simulink model "TEST2_Thermostat_Logic"  (R2025b)
settings: Solver=FixedStepAuto  StartTime=0.0  StopTime=60  FixedStep=0.1  RelTol=1e-3
settings Model: Creator=daniel.camacho  LastModifiedBy=daniel.camacho

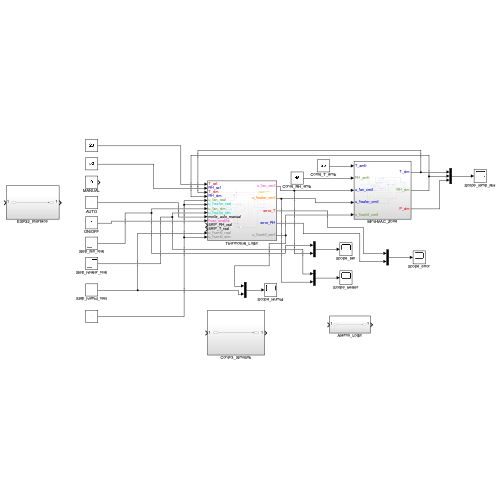
[thumbnail: Simulink's stored preview of the top-level diagram]
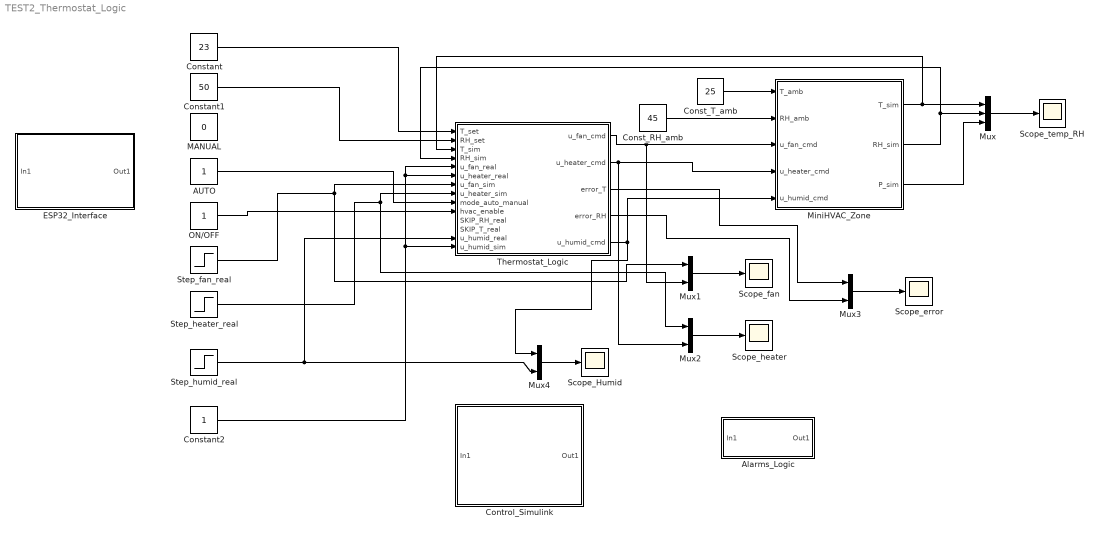
== system TEST2_Thermostat_Logic ==
  AUTO : Constant
  Alarms_Logic : Subsystem
  Const_RH_amb : Constant  Value=45
  Const_T_amb : Constant  Value=25
  Constant : Constant  Value=23
  Constant1 : Constant  Value=50
  Constant2 : Constant
  Control_Simulink : Subsystem
  ESP32_Interface : Subsystem
  MANUAL : Constant  Value=0
  MiniHVAC_Zone : Subsystem
  Mux : Mux  Inputs=3
  Mux{1..4} (4 alike) : Mux  Inputs=2
  ON/OFF : Constant
  Scope_Humid : Scope
      settings: ActiveDisplayYMinimum=-0.12499999999999997  ActiveDisplayYMaximum=1.125  DataLoggingVariableName=ScopeData3
  Scope_error : Scope
      settings: ActiveDisplayYMinimum=-2.875  ActiveDisplayYMaximum=5.875  DataLoggingVariableName=ScopeData4
  Scope_fan : Scope
      settings: ActiveDisplayYMinimum=-0.19683069160090955  ActiveDisplayYMaximum=1.476509953511558
  Scope_heater : Scope
      settings: ActiveDisplayYMinimum=-0.12499999999999997  ActiveDisplayYMaximum=1.125  DataLoggingVariableName=ScopeData2
  Scope_temp_RH : Scope
      settings: ActiveDisplayYMinimum=-1  ActiveDisplayYMaximum=1
  Step_fan_real : Step  Time=10  SampleTime=0
  Step_heater_real : Step  Time=20  SampleTime=0
  Step_humid_real : Step  Time=10  SampleTime=0
  Thermostat_Logic : Subsystem
  wires:
  Constant/1 -> Thermostat_Logic/1(T_set)
  Constant1/1 -> Thermostat_Logic/2(RH_set)
  ON/OFF/1 -> Thermostat_Logic/10(hvac_enable)
  Step_fan_real/1 -> Thermostat_Logic/7(u_fan_sim), Mux1/1
  Step_heater_real/1 -> Thermostat_Logic/8(u_heater_sim), Mux2/1
  Constant2/1 -> Thermostat_Logic/14(u_humid_sim), Thermostat_Logic/6(u_heater_real), Thermostat_Logic/5(u_fan_real)
  MiniHVAC_Zone/1(T_sim) -> Mux/1, Thermostat_Logic/3(T_sim)
  MiniHVAC_Zone/2(RH_sim) -> Mux/2, Thermostat_Logic/4(RH_sim)
  Thermostat_Logic/1(u_fan_cmd) -> MiniHVAC_Zone/3(u_fan_cmd), Mux1/2
  Thermostat_Logic/2(u_heater_cmd) -> MiniHVAC_Zone/4(u_heater_cmd), Mux2/2
  Const_T_amb/1 -> MiniHVAC_Zone/1(T_amb)
  Const_RH_amb/1 -> MiniHVAC_Zone/2(RH_amb)
  Mux/1 -> Scope_temp_RH/1
  MiniHVAC_Zone/3(P_sim) -> Mux/3
  Mux1/1 -> Scope_fan/1
  Mux2/1 -> Scope_heater/1
  Mux3/1 -> Scope_error/1
  Thermostat_Logic/3(error_T) -> Mux3/1
  Thermostat_Logic/4(error_RH) -> Mux3/2
  AUTO/1 -> Thermostat_Logic/9(mode_auto_manual)
  Mux4/1 -> Scope_Humid/1
  Step_humid_real/1 -> Thermostat_Logic/13(u_humid_real), Mux4/2
  Thermostat_Logic/5(u_humid_cmd) -> Mux4/1, MiniHVAC_Zone/5(u_humid_cmd)

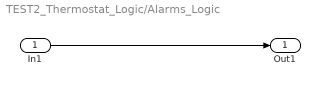
== system TEST2_Thermostat_Logic/Alarms_Logic ==
  In1 : Inport
  Out1 : Outport
  wires:
  In1/1 -> Out1/1

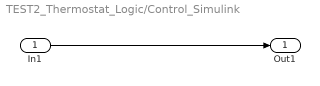
== system TEST2_Thermostat_Logic/Control_Simulink ==
  In1 : Inport
  Out1 : Outport
  wires:
  In1/1 -> Out1/1

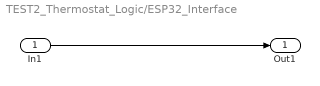
== system TEST2_Thermostat_Logic/ESP32_Interface ==
  In1 : Inport
  Out1 : Outport
  wires:
  In1/1 -> Out1/1

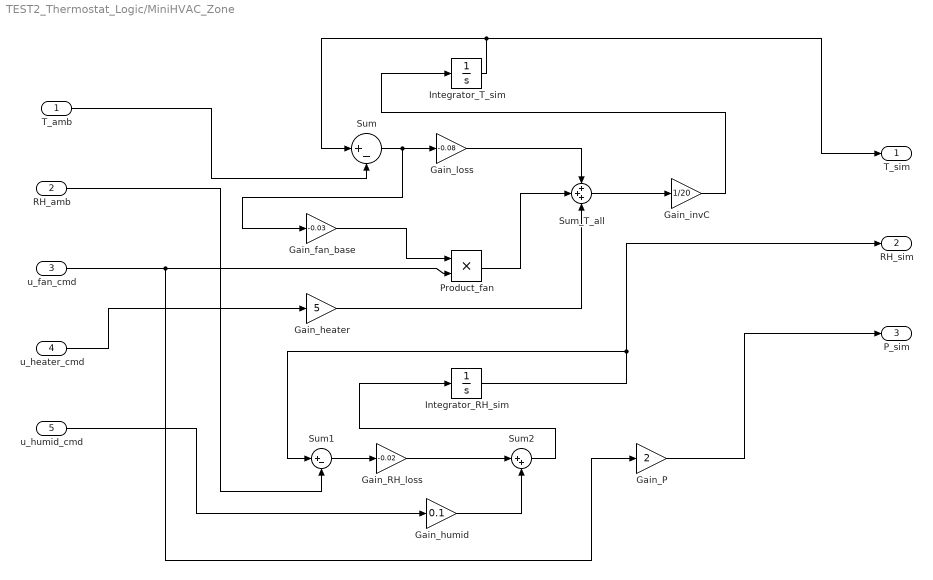
== system TEST2_Thermostat_Logic/MiniHVAC_Zone ==
  T_amb : Inport
  RH_amb : Inport  Port=2
  u_fan_cmd : Inport  Port=3
  u_heater_cmd : Inport  Port=4
  u_humid_cmd : Inport  Port=5
  Gain_P : Gain  Gain=2
  Gain_RH_loss : Gain  Gain=-0.02
  Gain_fan_base : Gain  Gain=-0.03
  Gain_heater : Gain  Gain=5
  Gain_humid : Gain  Gain=0.1
  Gain_invC : Gain  Gain=1/20
  Gain_loss : Gain  Gain=-0.08
  Integrator_RH_sim : Integrator  InitialCondition=45
  Integrator_T_sim : Integrator  InitialCondition=25
  Product_fan : Product
  Sum : Sum  Inputs=|+-
  Sum1 : Sum  Inputs=|+-
  Sum2 : Sum  Inputs=|++
  Sum_T_all : Sum  Inputs=+++
  T_sim : Outport
  RH_sim : Outport  Port=2
  P_sim : Outport  Port=3
  wires:
  Integrator_T_sim/1 -> T_sim/1, Sum/1
  T_amb/1 -> Sum/2
  Gain_fan_base/1 -> Product_fan/1
  u_fan_cmd/1 -> Gain_P/1, Product_fan/2
  u_heater_cmd/1 -> Gain_heater/1
  Sum/1 -> Gain_loss/1, Gain_fan_base/1
  Gain_loss/1 -> Sum_T_all/1
  Product_fan/1 -> Sum_T_all/2
  Gain_heater/1 -> Sum_T_all/3
  Sum_T_all/1 -> Gain_invC/1
  Gain_invC/1 -> Integrator_T_sim/1
  Integrator_RH_sim/1 -> RH_sim/1, Sum1/1
  RH_amb/1 -> Sum1/2
  Sum1/1 -> Gain_RH_loss/1
  u_humid_cmd/1 -> Gain_humid/1
  Gain_RH_loss/1 -> Sum2/1
  Gain_humid/1 -> Sum2/2
  Sum2/1 -> Integrator_RH_sim/1
  Gain_P/1 -> P_sim/1

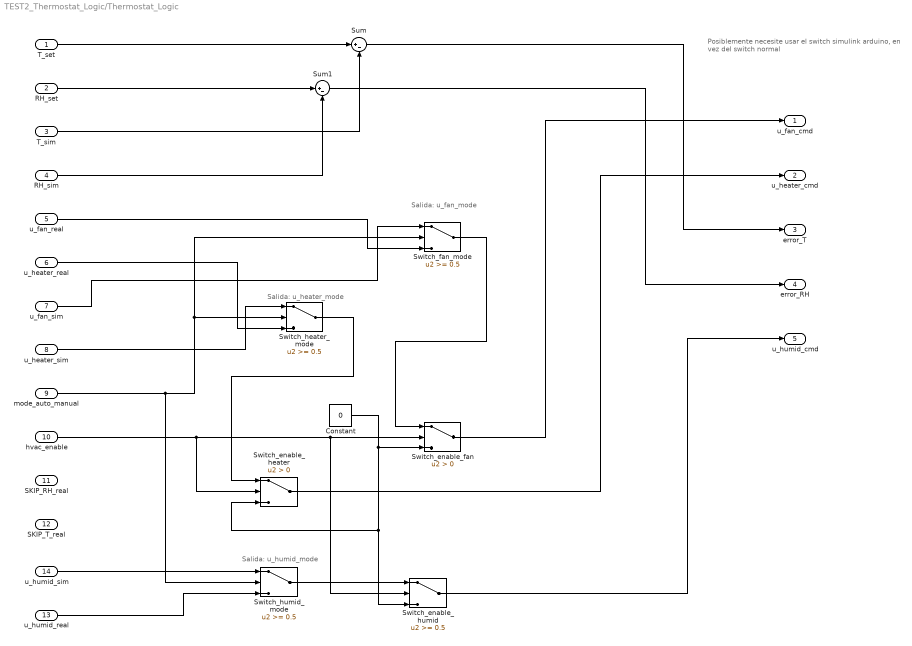
== system TEST2_Thermostat_Logic/Thermostat_Logic ==
  note: Salida: u_fan_mode
  note: Posiblemente necesite usar el switch simulink arduino,
      | en vez del switch normal
  note: Salida: u_heater_mode
  note: Salida: u_humid_mode
  T_set : Inport
  RH_set : Inport  Port=2
  T_sim : Inport  Port=3
  RH_sim : Inport  Port=4
  u_fan_real : Inport  Port=5
  u_heater_real : Inport  Port=6
  u_fan_sim : Inport  Port=7
  u_heater_sim : Inport  Port=8
  mode_auto_manual : Inport  Port=9
  hvac_enable : Inport  Port=10
  SKIP_RH_real : Inport  Port=11
  SKIP_T_real : Inport  Port=12
  u_humid_real : Inport  Port=13
  u_humid_sim : Inport  Port=14
  Constant : Constant  Value=0
  Sum : Sum  Inputs=|+-
  Sum1 : Sum  Inputs=|+-
  Switch_enable_fan : Switch  Criteria=u2 > Threshold  SaturateOnIntegerOverflow=off  InputSameDT=off
  Switch_enable_heater : Switch  Criteria=u2 > Threshold  SaturateOnIntegerOverflow=off  InputSameDT=off
  Switch_enable_humid : Switch  Threshold=0.5  SaturateOnIntegerOverflow=off  InputSameDT=off
  Switch_fan_mode : Switch  Threshold=0.5  SaturateOnIntegerOverflow=off  InputSameDT=off
  Switch_heater_mode : Switch  Threshold=0.5  OutMin=0  OutMax=1  SaturateOnIntegerOverflow=off  InputSameDT=off
  Switch_humid_mode : Switch  Threshold=0.5  SaturateOnIntegerOverflow=off  InputSameDT=off
  u_fan_cmd : Outport
  u_heater_cmd : Outport  Port=2
  error_T : Outport  Port=3
  error_RH : Outport  Port=4
  u_humid_cmd : Outport  Port=5
  wires:
  T_set/1 -> Sum/1
  T_sim/1 -> Sum/2
  Sum/1 -> error_T/1
  RH_set/1 -> Sum1/1
  RH_sim/1 -> Sum1/2
  Sum1/1 -> error_RH/1
  Switch_enable_fan/1 -> u_fan_cmd/1
  Switch_enable_heater/1 -> u_heater_cmd/1
  u_fan_real/1 -> Switch_fan_mode/3
  u_fan_sim/1 -> Switch_fan_mode/1
  u_heater_sim/1 -> Switch_heater_mode/1
  u_heater_real/1 -> Switch_heater_mode/3
  Switch_fan_mode/1 -> Switch_enable_fan/1
  Switch_heater_mode/1 -> Switch_enable_heater/1
  u_humid_sim/1 -> Switch_humid_mode/1
  Switch_enable_humid/1 -> u_humid_cmd/1
  mode_auto_manual/1 -> Switch_fan_mode/2, Switch_heater_mode/2, Switch_humid_mode/2
  Switch_humid_mode/1 -> Switch_enable_humid/1
  u_humid_real/1 -> Switch_humid_mode/3
  hvac_enable/1 -> Switch_enable_humid/2, Switch_enable_fan/2, Switch_enable_heater/2
  Constant/1 -> Switch_enable_fan/3, Switch_enable_humid/3, Switch_enable_heater/3
